simulink model "SF_cs_st2"  (R2024b)
settings: Solver=VariableStepAuto  StartTime=0.0  StopTime=10.0  RelTol=1e-3
libraries: spsFourierLib x1
settings Model: Creator=potat  LastModifiedBy=potat

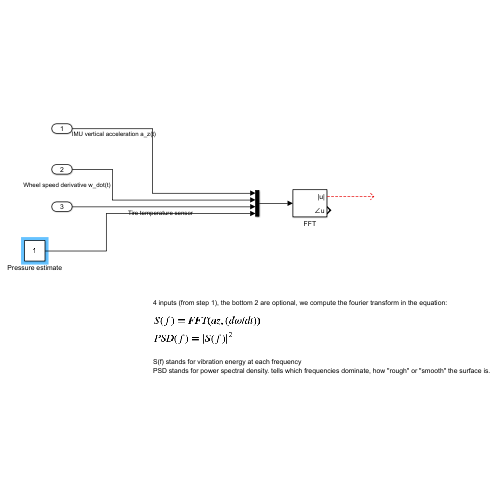
[thumbnail: Simulink's stored preview of the top-level diagram]
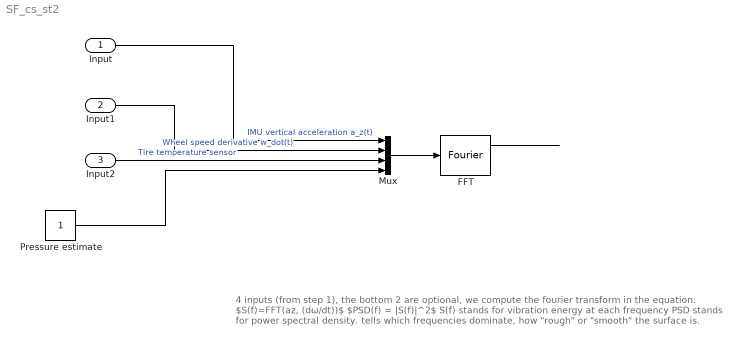
== system SF_cs_st2 ==
  note: 4 inputs (from step 1), the bottom 2 are optional, we compute the fourier transform in the equation:
      |
      | $S(f)=FFT(az​, (dω/dt))$
      | $PSD(f) = |S(f)|^2$
      |
      | S(f) stands for vibration energy at each frequency
      | PSD stands for power spectral density. tells which frequencies dominate, how "rough" or "smooth" the surface is.
  Input : Inport
  Input1 : Inport  Port=2
  Input2 : Inport  Port=3
  FFT : spsFourierLib/Fourier  Freq=60  n=1  InInit=[0, 0]  Ts=0
  Mux : Mux
  Pressure estimate : Constant
  wires:
  Input/1 -> Mux/1  "IMU vertical acceleration a_z(t)"
  Input1/1 -> Mux/2  "Wheel speed derivative w_dot(t)"
  Input2/1 -> Mux/3  "Tire temperature sensor"
  Pressure estimate/1 -> Mux/4
  Mux/1 -> FFT/1
  FFT/1 -> ?
